simulink model "model"  (Simulink 7.7)
settings: Solver=FixedStepDiscrete  StartTime=0.0  StopTime=2e2  FixedStep=T0  RelTol=1e-3
values from neighbouring files (symbols this model uses):
  P = conv(Bplus,P1)    [dalin_nomin.m]    (also in main.m = tmp(2:end); prefilter.m = 1)
  Q = [koef*Ad zeros(1,d)]    [dalin_nomin.m]    (also in main.m = 1000*eye(n))
  T0 = 1    [main.m]
libraries: cstblocks x1
settings Model: Creator=Administrator  LastModifiedBy=melanholly

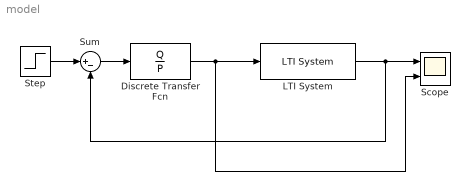
== system model ==
  Discrete Transfer Fcn : DiscreteTransferFcn  Numerator=Q  Denominator=P  SampleTime=T0
  LTI System : cstblocks/LTI System  SystemSampleTime=-1  sys=Wd  IC=[]
  Scope : Scope  NumInputPorts=2
      settings: TimeRange=150  YMin=0~-0.2  YMax=1.6~0.7
  Step : Step  SampleTime=T0
  Sum : Sum  Inputs=|+-
  wires:
  Step/1 -> Sum/1
  Sum/1 -> Discrete Transfer Fcn/1
  LTI System/1 -> Scope/1, Sum/2
  Discrete Transfer Fcn/1 -> LTI System/1, Scope/2
